simulink model "Low_pass_filter"  (R2016b)
settings: Solver=ode4  StartTime=0.0  StopTime=t(end)  FixedStep=0.01  RelTol=1e-3
settings Model: Creator=Testrechner  LastModifiedBy=Testrechner

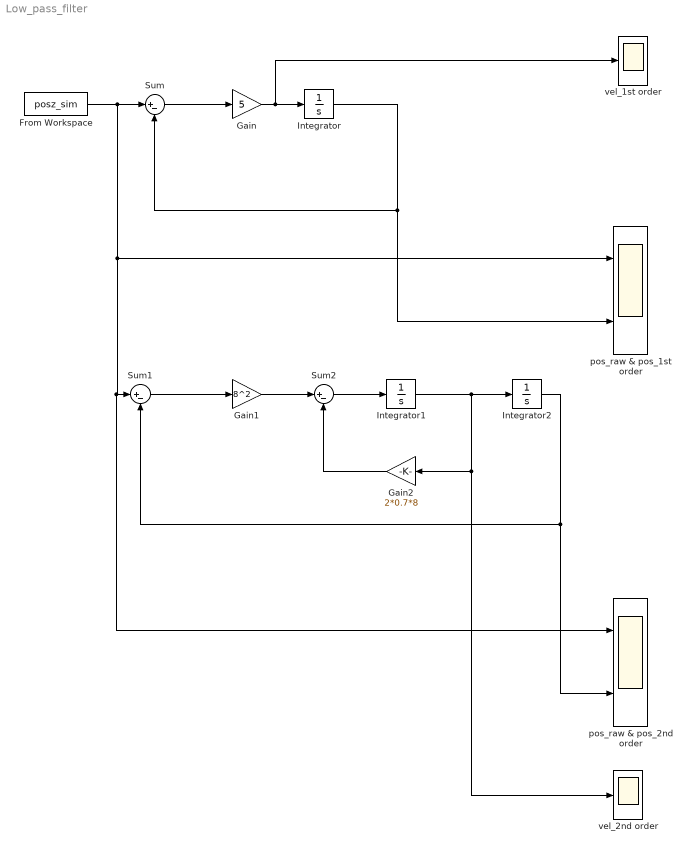
== system Low_pass_filter ==
  From Workspace : FromWorkspace  VariableName=posz_sim  SampleTime=0.01
  Gain : Gain  Gain=5
  Gain1 : Gain  Gain=8^2
  Gain2 : Gain  Gain=2*0.7*8
  Integrator : Integrator
  Integrator1 : Integrator
  Integrator2 : Integrator
  Sum : Sum  Inputs=|+-
  Sum1 : Sum  Inputs=|+-
  Sum2 : Sum  Inputs=|+-
  pos_raw & pos_1st order : Scope  NumInputPorts=2
  pos_raw & pos_2nd order : Scope  NumInputPorts=2
  vel_1st order : Scope
  vel_2nd order : Scope
  wires:
  From Workspace/1 -> pos_raw & pos_1st order/1, pos_raw & pos_2nd order/1, Sum1/1, Sum/1
  Sum/1 -> Gain/1
  Gain/1 -> vel_1st order/1, Integrator/1
  Integrator/1 -> Sum/2, pos_raw & pos_1st order/2
  Sum1/1 -> Gain1/1
  Gain1/1 -> Sum2/1
  Sum2/1 -> Integrator1/1
  Integrator1/1 -> Integrator2/1, vel_2nd order/1, Gain2/1
  Gain2/1 -> Sum2/2
  Integrator2/1 -> pos_raw & pos_2nd order/2, Sum1/2
